simulink model "liner"  (R2018b)
settings: Solver=VariableStepAuto  StartTime=0.0  StopTime=160  RelTol=1e-3
libraries: dsparch4 x4, commblkcod2 x2, commsink2 x2, commchan3 x1
settings Model: Creator=lance  LastModifiedBy=lance

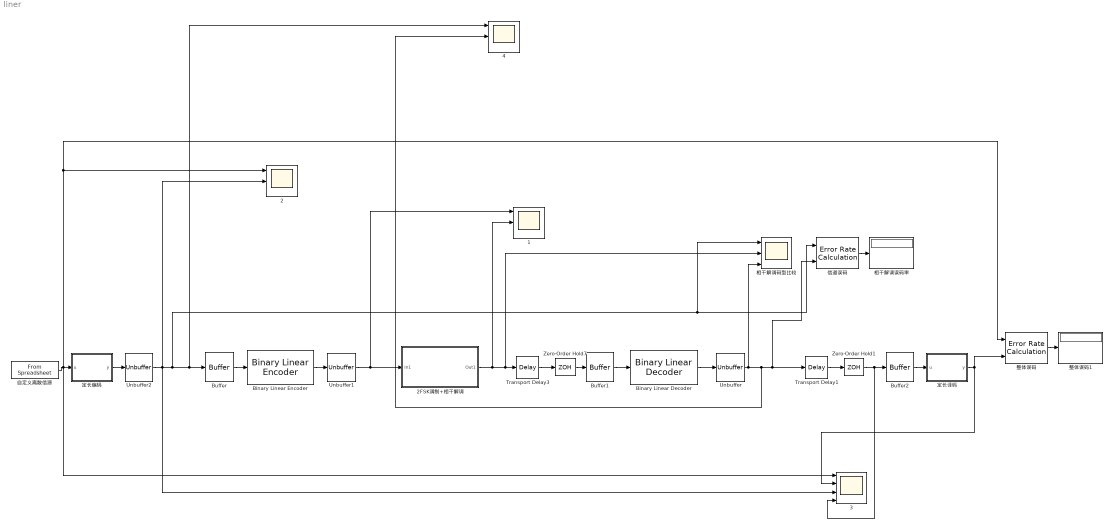
== system liner ==
  1 : Scope  NumInputPorts=3
  2 : Scope  NumInputPorts=3
  "2FSK调制+相干解调 " : Subsystem
  3 : Scope  NumInputPorts=4
  4 : Scope  NumInputPorts=3
  Binary Linear Decoder : commblkcod2/Binary Linear Decoder  G=[[1 1 0; 1 1 1;1 0 1] eye(3)]  trt=0
      settings: SourceProductName=Communications System Toolbox  SourceProductBaseCode=CM
  Binary Linear Encoder : commblkcod2/Binary Linear Encoder  G=[[1 1 0; 1 1 1; 1 0 1] eye(3)]
      settings: SourceProductName=Communications System Toolbox  SourceProductBaseCode=CM
  Buffer : Buffer  N=3  OutputFrames=off
  Buffer1 : Buffer  N=6  OutputFrames=off
  Buffer2 : Buffer  N=2  OutputFrames=off
  Transport Delay1 : TransportDelay  DelayTime=0.4
  Transport Delay3 : TransportDelay  DelayTime=0.8
  Unbuffer : Unbuffer
  Unbuffer1 : Unbuffer
  Unbuffer2 : Unbuffer
  Zero-Order Hold1 : ZeroOrderHold  SampleTime=0.4
  Zero-Order Hold7 : ZeroOrderHold  SampleTime=0.2
  "信道误码 " : commsink2/Error Rate Calculation  N=9  st_delay=0  cp_mode=Entire frame  subframe=[]  PMode=Port  WsName=ErrorVec  RsMode2=off  stop=off  numErr=100  maxBits=1e6
  定长编码 : MATLAB Function  TreatAsAtomicUnit=on
  "定长译码 " : MATLAB Function  TreatAsAtomicUnit=on
  整体误码 : commsink2/Error Rate Calculation  N=6  st_delay=0  cp_mode=Entire frame  subframe=[]  PMode=Port  WsName=ErrorVec  RsMode2=off  stop=off  numErr=100  maxBits=1e6
  "整体误码1 " : Display
  相干解调码型比较 : Scope  NumInputPorts=3
  相干解调误码率 : Display
  "自定义离散信源 " : FromSpreadsheet  FileName=C:\Users\lance\OneDrive\2020-2021-2\信息论\实验\1\s.xlsx  TreatFirstColumnAs=Data  SampleTime=0.8
  wires:
  "信道误码 "/1 -> 相干解调误码率/1
  "2FSK调制+相干解调 "/1(Out1) -> 1/2, Transport Delay3/1, 相干解调码型比较/2
  Binary Linear Encoder/1 -> Unbuffer1/1
  Buffer/1 -> Binary Linear Encoder/1
  Binary Linear Decoder/1 -> Unbuffer/1
  Unbuffer/1 -> 4/2, Transport Delay1/1, "信道误码 "/2, 相干解调码型比较/3
  Unbuffer1/1 -> 1/1, "2FSK调制+相干解调 "/1(In1)
  Buffer1/1 -> Binary Linear Decoder/1
  Transport Delay3/1 -> Zero-Order Hold7/1
  Zero-Order Hold7/1 -> Buffer1/1
  定长编码/1(y) -> Unbuffer2/1
  "自定义离散信源 "/1 -> 3/1, 2/1, 整体误码/1, 定长编码/1(u)
  Buffer2/1 -> "定长译码 "/1(u)
  Unbuffer2/1 -> 3/3, 2/2, "信道误码 "/1, 相干解调码型比较/1, 4/1, Buffer/1
  Transport Delay1/1 -> Zero-Order Hold1/1
  Zero-Order Hold1/1 -> 3/4, Buffer2/1
  "定长译码 "/1(y) -> 3/2, 整体误码/2
  整体误码/1 -> "整体误码1 "/1

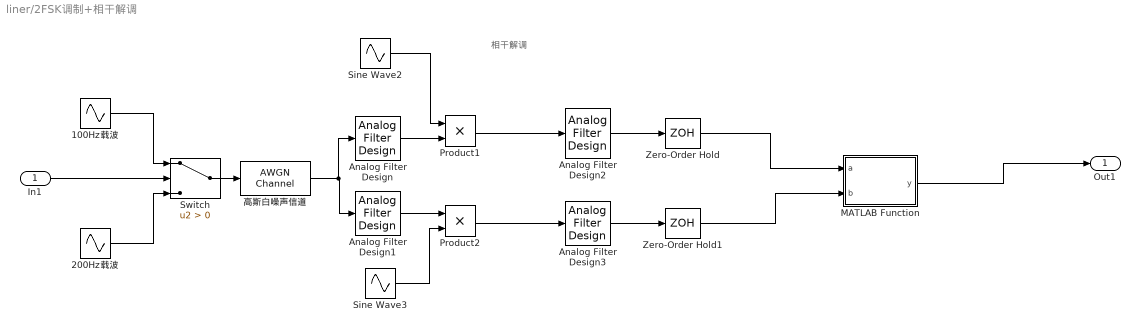
== system liner/2FSK调制+相干解调  ==
  note: 相干解调
  In1 : Inport
  100Hz载波 : Sin  Frequency=100*2*pi  SampleTime=0.0001
  200Hz载波 : Sin  Frequency=200*2*pi  SampleTime=0.0001
  Analog Filter Design : dsparch4/Analog Filter Design  method=Butterworth  filttype=Bandpass  N=8  Wlo=90*2*pi  Whi=110*2*pi  Rp=2  Rs=40
  Analog Filter Design1 : dsparch4/Analog Filter Design  method=Butterworth  filttype=Bandpass  N=8  Wlo=190*2*pi  Whi=210*2*pi  Rp=2  Rs=40
  Analog Filter Design2 : dsparch4/Analog Filter Design  method=Butterworth  filttype=Lowpass  N=8  Wlo=10*pi  Whi=103*2*pi  Rp=2  Rs=40
  Analog Filter Design3 : dsparch4/Analog Filter Design  method=Butterworth  filttype=Lowpass  N=8  Wlo=10*pi  Whi=103*2*pi  Rp=2  Rs=40
  MATLAB Function : MATLAB Function  TreatAsAtomicUnit=on
  Product1 : Product
  Product2 : Product
  Sine Wave2 : Sin  Frequency=100*2*pi  SampleTime=0.0001
  Sine Wave3 : Sin  Frequency=200*2*pi  SampleTime=0.0001
  Switch : Switch  Criteria=u2 > Threshold
  Zero-Order Hold : ZeroOrderHold  SampleTime=0.2
  Zero-Order Hold1 : ZeroOrderHold  SampleTime=0.2
  "高斯白噪声信道 " : commchan3/AWGN Channel  InputProcessing=Columns as channels (frame based)  seed=67  noiseMode="Signal to noise ratio  (SNR)"  EbNodB=1  EsNodB=10  SNRdB=-19  bitsPerSym=1  Ps=1  Tsym=1  variance=1
  Out1 : Outport
  wires:
  In1/1 -> Switch/2
  "高斯白噪声信道 "/1 -> Analog Filter Design1/1, Analog Filter Design/1
  Analog Filter Design3/1 -> Zero-Order Hold1/1
  100Hz载波/1 -> Switch/1
  Sine Wave3/1 -> Product2/2
  Switch/1 -> "高斯白噪声信道 "/1
  Product1/1 -> Analog Filter Design2/1
  Analog Filter Design/1 -> Product1/2
  200Hz载波/1 -> Switch/3
  Zero-Order Hold1/1 -> MATLAB Function/2(b)
  Sine Wave2/1 -> Product1/1
  Analog Filter Design2/1 -> Zero-Order Hold/1
  Zero-Order Hold/1 -> MATLAB Function/1(a)
  Analog Filter Design1/1 -> Product2/1
  Product2/1 -> Analog Filter Design3/1
  MATLAB Function/1(y) -> Out1/1

== matlab function liner/定长编码 ==
  data: y output; u input
function y = dingchangbianma(u)
switch u
    case 0
        y=[0;0];
    case 1
        y=[0;1];
    case 3
        y=[1;0];
    case 4
        y=[1;1];
    otherwise
        y=[1;1];
end

== matlab function liner/2FSK调制+相干解调 /MATLAB Function ==
  data: a input; y output; b input
function y = fcn(a, b)
if(a>b)
    y=1;
else
    y=0;
end

== matlab function liner/定长译码  ==
  data: u input; y output
function y = dingchangyima(u)
if u==[0;0]
    y=0;
elseif u==[0;1]
    y=1;
elseif u==[1;0]
    y=3;
else
    y=4;

end
